simulink model "SingleTrack"  (R2019b)
settings: Solver=ode1  StartTime=0  StopTime=250  FixedStep=1.0000000000000000e-003  RelTol=1e-3
InitFcn:
  | sampleTime = str2double(get_param(bdroot, 'FixedStep'));
undefined symbols (not defined in the file or in its folder): AccPedalPos, BrakePedalPos, BrakeSwitch, DiscIntNeverNeededParam, DYNA4, EngSpd, IgnitionSwitch, InitialGear, InitialSpeed, IntendedEngTrq, LeftIndicator, MainBrakePress, MaxGear, MDL, MinGear, RefAcc, RefLane, RefLatPos, RefPath, RefPathCurv, RefSpd, RefSpdPreview, RefSpdRetrospect, RightIndicator, SteeringWheelAng, SteeringWheelTrq, UserDefinedRefValue, vm_const
libraries: UtilitiesLibrary x31, simulink x18, WheelSystemModules x13, LongitudinalControllerModules x13, LateralControllerModules x7, AnimationBusselectorModules x5, EnvironmentModules x5, BasicEngineControlModules x5, MiscellaneousControlModules x5, Animation3Modules x4, AuxiliariesModules x4, ReducedTireModules x4
(part 3 of 32)

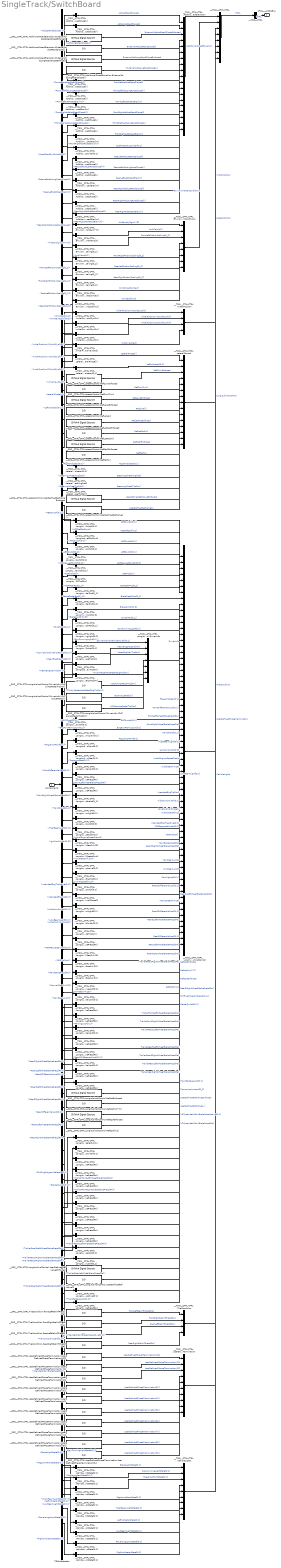
== system SingleTrack/SwitchBoard ==
  Components : Inport
  TDBusSelector : BusSelector  OutputSignals=Environment.AdditionalRoadElevation.AddLatRoadSlope[-],Environment.AdditionalRoadElevation.AddLongRoadSlope[-],Environment.AdditionalRoadElevation.FrontLeftAddLatRoadSlope[-],Environment.AdditionalRoadElevation.FrontLeftAddLongRoadSlope[-],Environment.AdditionalRoadElevation.FrontLeftAddRoadElev[m],Environment.AdditionalRoadElevation.FrontRightAddLatRoadSlope[-],Environment.AdditionalRoadElevation.FrontRightAddLongRoadSlope[-],Environment.AdditionalRoadElevation.FrontRightAddRoadElev[m],Environment.AdditionalRoadElevation.LocalRoadSysSwitch[0;1],Environment.AdditionalRoadElevation.RearLeftAddLatRoadSlope[-],Environment.AdditionalRoadElevation.RearLeftAddLongRoadSlope[-],Environment.AdditionalRoadElevation.RearLeftAddRoadElev[m],Environment.AdditionalRoadElevation.RearRightAddLatRoadSlope[-],Environment.AdditionalRoadElevation.RearRightAddLongRoadSlope[-],Environment.AdditionalRoadElevation.RearRightAddRoadElev[m],Environment.AmbientConditions.AirDensity[kg/m**3],Environment.AmbientConditions.AmbTemp[K],Environment.RoadFrictionScaling.FrontLeftFrictionScaling[0_2],Environment.RoadFrictionScaling.FrontRightFrictionScaling[0_2],Environment.RoadFrictionScaling.RearLeftFrictionScaling[0_2],Environment.RoadFrictionScaling.RearRightFrictionScaling[0_2],Environment.WindImpact.WindDirection[rad],Environment.WindImpact.WindSpd[m/s],VehicleControl.InitialConditions.InitialPositionX(WorldSys)[m],VehicleControl.InitialConditions.InitialPositionY(WorldSys)[m],VehicleControl.InitialConditions.InitialPositionZ(WorldSys)[m],VehicleControl.InitialConditions.InitialYaw[rad],VehicleControl.LateralControl.LateralPhase[-],VehicleControl.LateralControl.LeftIndicator[0;1],VehicleControl.LateralControl.RightIndicator[0;1],VehicleControl.LateralControl.SteeringWheelAng[rad],Vehicle.Chassis.FrontAxle.Steering.SteeringWheelTrq[Nm],VehicleControl.LongitudinalControl.ABSSwitch[0;1],VehicleControl.LongitudinalControl.ACCRefSpd[m/s],VehicleControl.LongitudinalControl.ACCSwitch[0;1],VehicleControl.LongitudinalControl.AEBSwitch[0;1],Vehicle.Drivetrain.DrivetrainControlUnit.TransmissionControlUnit.ASRRequestSwitch[0;2],Vehicle.Drivetrain.DrivetrainControlUnit.TransmissionControlUnit.ASRTrq[Nm],VehicleControl.LongitudinalControl.AccPedalPos[0_1],VehicleControl.LongitudinalControl.BrakePedalPos[0_1],VehicleControl.LongitudinalControl.BrakeSwitch[1;3],VehicleControl.LongitudinalControl.ClutchPos[0_1],VehicleControl.LongitudinalControl.DayRunningLight[0;1],ControlUnits.VCU.DriverInfo.ConventionalVehicleSwitch[0;1],Vehicle.Engine.EnginePhysics.Mechanics.MeanEngDragTrq[Nm],Vehicle.Engine.EnginePhysics.Mechanics.MeanEngMaxTrq[Nm],Vehicle.Engine.EnginePhysics.Mechanics.ThirtyPercentAccPedalEngTrq[Nm],VehicleControl.LongitudinalControl.ESCSwitch[0;1],ControlUnits.VCU.EngRunPermission[0;1],VehicleControl.LongitudinalControl.FogLampFront[0;1],VehicleControl.LongitudinalControl.FogLampRear[0;1],VehicleControl.LongitudinalControl.FrontDifferentialLock[0;1],VehicleControl.LongitudinalControl.FrontLeftWheelBrakePress[Pa],VehicleControl.LongitudinalControl.FrontRightWheelBrakePress[Pa],VehicleControl.LongitudinalControl.Handbrake[0_1],VehicleControl.LongitudinalControl.HighBeamLight[0;1],VehicleControl.LongitudinalControl.IgnitionSwitch[0;3],VehicleControl.LongitudinalControl.InitialEngineSpeed[rad/s],VehicleControl.LongitudinalControl.InitialGear[-4;20],VehicleControl.LongitudinalControl.InitialSpeed[m/s],ControlUnits.VCU.IntendedEngTrqActive[0;1],ControlUnits.VCU.IntendedEngTrq[Nm],VehicleControl.LongitudinalControl.KickdownSwitch[0;1],VehicleControl.LongitudinalControl.LongitudinalPhase[-],VehicleControl.LongitudinalControl.LowBeamLight[0;1],Vehicle.Drivetrain.DrivetrainControlUnit.TransmissionControlUnit.MSRRequestSwitch[0;2],Vehicle.Drivetrain.DrivetrainControlUnit.TransmissionControlUnit.MSRTrq[Nm],VehicleControl.LongitudinalControl.MainBrakePress[Pa],VehicleControl.LongitudinalControl.ManualGear[-4;20],VehicleControl.LongitudinalControl.AutomaticGearRange.MaxGear[-4;20],VehicleControl.LongitudinalControl.AutomaticGearRange.MinGear[-4;20],VehicleControl.LongitudinalControl.ParkingLock[0;1],VehicleControl.LongitudinalControl.Rear2DifferentialLock[0;1],VehicleControl.LongitudinalControl.Rear2LeftWheelBrakePress[Pa],VehicleControl.LongitudinalControl.Rear2RightWheelBrakePress[Pa],VehicleControl.LongitudinalControl.Rear3DifferentialLock[0;1],VehicleControl.LongitudinalControl.Rear3LeftWheelBrakePress[Pa],VehicleControl.LongitudinalControl.Rear3RightWheelBrakePress[Pa],VehicleControl.LongitudinalControl.RearDifferentialLock[0;1],VehicleControl.LongitudinalControl.RearLeftWheelBrakePress[Pa],VehicleControl.LongitudinalControl.RearRightWheelBrakePress[Pa],VehicleControl.LongitudinalControl.ShiftingProgramSelection[-],Vehicle.Engine.EngineControlUnit.StarterSwitch[0;1],VehicleControl.LongitudinalControl.TrailerFrontLeftWheelBrakePress[Pa],VehicleControl.LongitudinalControl.TrailerFrontRightWheelBrakePress[Pa],VehicleControl.LongitudinalControl.TrailerRear2LeftWheelBrakePress[Pa],VehicleControl.LongitudinalControl.TrailerRear2RightWheelBrakePress[Pa],VehicleControl.LongitudinalControl.TrailerRear3LeftWheelBrakePress[Pa],VehicleControl.LongitudinalControl.TrailerRear3RightWheelBrakePress[Pa],VehicleControl.LongitudinalControl.TrailerRearLeftWheelBrakePress[Pa],VehicleControl.LongitudinalControl.TrailerRearRightWheelBrakePress[Pa],VehicleControl.LongitudinalControl.TransferCaseLock[0;1],ControlUnits.VCU.TransmissionLoad[0_1],ControlUnits.VCU.IntendedMainBrakePressActive[0;1],ControlUnits.VCU.IntendedMainBrakePress[Pa],ControlUnits.LCU.VehicleLights.BrakeLightState[0;1],ControlUnits.LCU.VehicleLights.DayRunningLightState[0;1],ControlUnits.LCU.VehicleLights.FogLampFrontState[0;1],ControlUnits.LCU.VehicleLights.FogLampRearState[0;1],ControlUnits.LCU.VehicleLights.HighBeamLightState[0;1],ControlUnits.LCU.VehicleLights.LeftIndicatorState[0;1],ControlUnits.LCU.VehicleLights.LowBeamLightState[0;1],ControlUnits.LCU.VehicleLights.ReversingLampState[0;1],ControlUnits.LCU.VehicleLights.RightIndicatorState[0;1]
  __SRC__CTRL.CTRL.AdditionalRoadElevation.ExternalAddLatRoadSlopeEnforced : UtilitiesLibrary/DYNA4 Signal Source  Tag=DYNA4_Signal_Source  accessId=DYNA4.ModelHandling.AccessID.format('CTRL.AdditionalRoadElevation.ExternalAddLatRoadSlopeEnforced', 'parentId', parentId, 'blockName', blockName)  initialValue=0.0  sampleTime=sampleTime
  __SRC__CTRL.CTRL.AdditionalRoadElevation.ExternalAddLatRoadSlope[-] : Constant  Value=0.0  OutDataTypeStr=Inherit: Inherit via back propagation
  __SRC__CTRL.CTRL.AdditionalRoadElevation.ExternalAddLongRoadSlopeEnforced : UtilitiesLibrary/DYNA4 Signal Source  Tag=DYNA4_Signal_Source  accessId=DYNA4.ModelHandling.AccessID.format('CTRL.AdditionalRoadElevation.ExternalAddLongRoadSlopeEnforced', 'parentId', parentId, 'blockName', blockName)  initialValue=0.0  sampleTime=sampleTime
  __SRC__CTRL.CTRL.AdditionalRoadElevation.ExternalAddLongRoadSlope[-] : Constant  Value=0.0  OutDataTypeStr=Inherit: Inherit via back propagation
  __SRC__CTRL.CTRL.LateralControl.RefCurvEnforced : UtilitiesLibrary/DYNA4 Signal Source  Tag=DYNA4_Signal_Source  accessId=DYNA4.ModelHandling.AccessID.format('CTRL.LateralControl.RefCurvEnforced', 'parentId', parentId, 'blockName', blockName)  initialValue=0.0  sampleTime=sampleTime
  __SRC__CTRL.CTRL.LateralControl.RefCurv[1/m] : Constant  Value=0.0  OutDataTypeStr=Inherit: Inherit via back propagation
  __SRC__CTRL.CTRL.LateralControl.RefLaneEnforced : UtilitiesLibrary/DYNA4 Signal Source  Tag=DYNA4_Signal_Source  accessId=DYNA4.ModelHandling.AccessID.format('CTRL.LateralControl.RefLaneEnforced', 'parentId', parentId, 'blockName', blockName)  initialValue=0.0  sampleTime=sampleTime
  __SRC__CTRL.CTRL.LateralControl.RefLane[-] : Constant  Value=0.0  OutDataTypeStr=Inherit: Inherit via back propagation
  __SRC__CTRL.CTRL.LateralControl.RefLatPosEnforced : UtilitiesLibrary/DYNA4 Signal Source  Tag=DYNA4_Signal_Source  accessId=DYNA4.ModelHandling.AccessID.format('CTRL.LateralControl.RefLatPosEnforced', 'parentId', parentId, 'blockName', blockName)  initialValue=0.0  sampleTime=sampleTime
  __SRC__CTRL.CTRL.LateralControl.RefLatPos[m] : Constant  Value=0.0  OutDataTypeStr=Inherit: Inherit via back propagation
  __SRC__CTRL.CTRL.LateralControl.RefPathEnforced : UtilitiesLibrary/DYNA4 Signal Source  Tag=DYNA4_Signal_Source  accessId=DYNA4.ModelHandling.AccessID.format('CTRL.LateralControl.RefPathEnforced', 'parentId', parentId, 'blockName', blockName)  initialValue=0.0  sampleTime=sampleTime
  __SRC__CTRL.CTRL.LateralControl.RefPath[-] : Constant  Value=0.0  OutDataTypeStr=Inherit: Inherit via back propagation
  __SRC__CTRL.CTRL.LateralControl.UserDefinedRefValueEnforced : UtilitiesLibrary/DYNA4 Signal Source  Tag=DYNA4_Signal_Source  accessId=DYNA4.ModelHandling.AccessID.format('CTRL.LateralControl.UserDefinedRefValueEnforced', 'parentId', parentId, 'blockName', blockName)  initialValue=0.0  sampleTime=sampleTime
  __SRC__CTRL.CTRL.LateralControl.UserDefinedRefValue[-] : Constant  Value=0.0  OutDataTypeStr=Inherit: Inherit via back propagation
  __SRC__CTRL.CTRL.LongitudinalControl.DriverInfo.VCUFullAccPedalTrq[Nm] : Constant  Value=0.0  OutDataTypeStr=Inherit: Inherit via back propagation
  __SRC__CTRL.CTRL.LongitudinalControl.DriverInfo.VCUTorqueRatio[-] : Constant  Value=0.0  OutDataTypeStr=Inherit: Inherit via back propagation
  __SRC__CTRL.CTRL.LongitudinalControl.DriverInfo.VCUZeroAccPedalTrq[Nm] : Constant  Value=0.0  OutDataTypeStr=Inherit: Inherit via back propagation
  __SRC__CTRL.CTRL.LongitudinalControl.RefAccEnforced : UtilitiesLibrary/DYNA4 Signal Source  Tag=DYNA4_Signal_Source  accessId=DYNA4.ModelHandling.AccessID.format('CTRL.LongitudinalControl.RefAccEnforced', 'parentId', parentId, 'blockName', blockName)  initialValue=0.0  sampleTime=sampleTime
  __SRC__CTRL.CTRL.LongitudinalControl.RefAcc[m/s**2] : Constant  Value=0.0  OutDataTypeStr=Inherit: Inherit via back propagation
  __SRC__CTRL.CTRL.LongitudinalControl.RefSpdEnforced : UtilitiesLibrary/DYNA4 Signal Source  Tag=DYNA4_Signal_Source  accessId=DYNA4.ModelHandling.AccessID.format('CTRL.LongitudinalControl.RefSpdEnforced', 'parentId', parentId, 'blockName', blockName)  initialValue=0.0  sampleTime=sampleTime
  __SRC__CTRL.CTRL.LongitudinalControl.RefSpd[m/s] : Constant  Value=0.0  OutDataTypeStr=Inherit: Inherit via back propagation
  __SRC__CTRL.CTRL.LongitudinalControl.UserDefinedRefValueEnforced : UtilitiesLibrary/DYNA4 Signal Source  Tag=DYNA4_Signal_Source  accessId=DYNA4.ModelHandling.AccessID.format('CTRL.LongitudinalControl.UserDefinedRefValueEnforced', 'parentId', parentId, 'blockName', blockName)  initialValue=0.0  sampleTime=sampleTime
  __SRC__CTRL.CTRL.LongitudinalControl.UserDefinedRefValue[-] : Constant  Value=0.0  OutDataTypeStr=Inherit: Inherit via back propagation
  __SRC__CTRL.CTRL.TireCondition.FrontLeftRelInflPress[Pa] : Constant  Value=0.0  OutDataTypeStr=Inherit: Inherit via back propagation
  __SRC__CTRL.CTRL.TireCondition.FrontRightRelInflPress[Pa] : Constant  Value=0.0  OutDataTypeStr=Inherit: Inherit via back propagation
  __SRC__CTRL.CTRL.TireCondition.RearLeftRelInflPress[Pa] : Constant  Value=0.0  OutDataTypeStr=Inherit: Inherit via back propagation
  __SRC__CTRL.CTRL.TireCondition.RearRightRelInflPress[Pa] : Constant  Value=0.0  OutDataTypeStr=Inherit: Inherit via back propagation
  __SRC__CTRL.CTRL.UserDefinedPhaseTermination.UserDefinedPhaseTermination10[-] : Constant  Value=0.0  OutDataTypeStr=Inherit: Inherit via back propagation
  __SRC__CTRL.CTRL.UserDefinedPhaseTermination.UserDefinedPhaseTermination1[-] : Constant  Value=0.0  OutDataTypeStr=Inherit: Inherit via back propagation
  __SRC__CTRL.CTRL.UserDefinedPhaseTermination.UserDefinedPhaseTermination2[-] : Constant  Value=0.0  OutDataTypeStr=Inherit: Inherit via back propagation
  __SRC__CTRL.CTRL.UserDefinedPhaseTermination.UserDefinedPhaseTermination3[-] : Constant  Value=0.0  OutDataTypeStr=Inherit: Inherit via back propagation
  __SRC__CTRL.CTRL.UserDefinedPhaseTermination.UserDefinedPhaseTermination4[-] : Constant  Value=0.0  OutDataTypeStr=Inherit: Inherit via back propagation
  __SRC__CTRL.CTRL.UserDefinedPhaseTermination.UserDefinedPhaseTermination5[-] : Constant  Value=0.0  OutDataTypeStr=Inherit: Inherit via back propagation
  __SRC__CTRL.CTRL.UserDefinedPhaseTermination.UserDefinedPhaseTermination6[-] : Constant  Value=0.0  OutDataTypeStr=Inherit: Inherit via back propagation
  __SRC__CTRL.CTRL.UserDefinedPhaseTermination.UserDefinedPhaseTermination7[-] : Constant  Value=0.0  OutDataTypeStr=Inherit: Inherit via back propagation
  __SRC__CTRL.CTRL.UserDefinedPhaseTermination.UserDefinedPhaseTermination8[-] : Constant  Value=0.0  OutDataTypeStr=Inherit: Inherit via back propagation
  __SRC__CTRL.CTRL.UserDefinedPhaseTermination.UserDefinedPhaseTermination9[-] : Constant  Value=0.0  OutDataTypeStr=Inherit: Inherit via back propagation
  __TDD__CTRL.CTRL.AdditionalRoadElevation.AddLatRoadSlope[-] : Demux  Outputs=[1]
  __TDD__CTRL.CTRL.AdditionalRoadElevation.AddLongRoadSlope[-] : Demux  Outputs=[1]
  __TDD__CTRL.CTRL.AdditionalRoadElevation.FrontLeftAddLatRoadSlope[-] : Demux  Outputs=[1]
  __TDD__CTRL.CTRL.AdditionalRoadElevation.FrontLeftAddLongRoadSlope[-] : Demux  Outputs=[1]
  __TDD__CTRL.CTRL.AdditionalRoadElevation.FrontLeftAddRoadElev[m] : Demux  Outputs=[1]
  __TDD__CTRL.CTRL.AdditionalRoadElevation.FrontRightAddLatRoadSlope[-] : Demux  Outputs=[1]
  __TDD__CTRL.CTRL.AdditionalRoadElevation.FrontRightAddLongRoadSlope[-] : Demux  Outputs=[1]
  __TDD__CTRL.CTRL.AdditionalRoadElevation.FrontRightAddRoadElev[m] : Demux  Outputs=[1]
  __TDD__CTRL.CTRL.AdditionalRoadElevation.LocalRoadSysSwitch[0;1] : Demux  Outputs=[1]
  __TDD__CTRL.CTRL.AdditionalRoadElevation.RearLeftAddLatRoadSlope[-] : Demux  Outputs=[1]
  __TDD__CTRL.CTRL.AdditionalRoadElevation.RearLeftAddLongRoadSlope[-] : Demux  Outputs=[1]
  __TDD__CTRL.CTRL.AdditionalRoadElevation.RearLeftAddRoadElev[m] : Demux  Outputs=[1]
  __TDD__CTRL.CTRL.AdditionalRoadElevation.RearRightAddLatRoadSlope[-] : Demux  Outputs=[1]
  __TDD__CTRL.CTRL.AdditionalRoadElevation.RearRightAddLongRoadSlope[-] : Demux  Outputs=[1]
  __TDD__CTRL.CTRL.AdditionalRoadElevation.RearRightAddRoadElev[m] : Demux  Outputs=[1]
  __TDD__CTRL.CTRL.EnvironmentalConditions.AirDensity[kg/m**3] : Demux  Outputs=[1]
  __TDD__CTRL.CTRL.EnvironmentalConditions.AmbTemp[K] : Demux  Outputs=[1]
  __TDD__CTRL.CTRL.EnvironmentalConditions.FrontLeftFrictionScaling[0_2] : Demux  Outputs=[1]
  __TDD__CTRL.CTRL.EnvironmentalConditions.FrontRightFrictionScaling[0_2] : Demux  Outputs=[1]
  __TDD__CTRL.CTRL.EnvironmentalConditions.RearLeftFrictionScaling[0_2] : Demux  Outputs=[1]
  __TDD__CTRL.CTRL.EnvironmentalConditions.RearRightFrictionScaling[0_2] : Demux  Outputs=[1]
  __TDD__CTRL.CTRL.EnvironmentalConditions.WindDirection[rad] : Demux  Outputs=[1]
  __TDD__CTRL.CTRL.EnvironmentalConditions.WindSpd[m/s] : Demux  Outputs=[1]
  __TDD__CTRL.CTRL.InitialPosition.InitialPositionX(WorldSys)[m] : Demux  Outputs=[1]
  __TDD__CTRL.CTRL.InitialPosition.InitialPositionY(WorldSys)[m] : Demux  Outputs=[1]
  __TDD__CTRL.CTRL.InitialPosition.InitialPositionZ(WorldSys)[m] : Demux  Outputs=[1]
  __TDD__CTRL.CTRL.InitialPosition.InitialYaw[rad] : Demux  Outputs=[1]
  __TDD__CTRL.CTRL.LateralControl.LateralPhase[-] : Demux  Outputs=1
  __TDD__CTRL.CTRL.LateralControl.LeftIndicator[0;1] : Demux  Outputs=[1]
  __TDD__CTRL.CTRL.LateralControl.RightIndicator[0;1] : Demux  Outputs=[1]
  __TDD__CTRL.CTRL.LateralControl.SteeringWheelAng[rad] : Demux  Outputs=[1]
  __TDD__CTRL.CTRL.LateralControl.SteeringWheelTrq[Nm] : Demux  Outputs=[1]
  __TDD__CTRL.CTRL.LongitudinalControl.ABSSwitch[0;1] : Demux  Outputs=[1]
  __TDD__CTRL.CTRL.LongitudinalControl.ACCRefSpd[m/s] : Demux  Outputs=[1]
  __TDD__CTRL.CTRL.LongitudinalControl.ACCSwitch[0;1] : Demux  Outputs=[1]
  __TDD__CTRL.CTRL.LongitudinalControl.AEBSwitch[0;1] : Demux  Outputs=[1]
  __TDD__CTRL.CTRL.LongitudinalControl.ASRRequestSwitch[0;2] : Demux  Outputs=1
  __TDD__CTRL.CTRL.LongitudinalControl.ASRTrq[Nm] : Demux  Outputs=1
  __TDD__CTRL.CTRL.LongitudinalControl.AccPedalPos[0_1] : Demux  Outputs=[1]
  __TDD__CTRL.CTRL.LongitudinalControl.BrakePedalPos[0_1] : Demux  Outputs=1
  __TDD__CTRL.CTRL.LongitudinalControl.BrakeSwitch[1;3] : Demux  Outputs=1
  __TDD__CTRL.CTRL.LongitudinalControl.ClutchPos[0_1] : Demux  Outputs=[1]
  __TDD__CTRL.CTRL.LongitudinalControl.DayRunningLight[0;1] : Demux  Outputs=[1]
  __TDD__CTRL.CTRL.LongitudinalControl.DriverInfo.ConventionalVehicleSwitch[0;1] : Demux  Outputs=[1]
  __TDD__CTRL.CTRL.LongitudinalControl.DriverInfo.MeanEngDragTrq[Nm] : Demux  Outputs=[1]
  __TDD__CTRL.CTRL.LongitudinalControl.DriverInfo.MeanEngMaxTrq[Nm] : Demux  Outputs=[1]
  __TDD__CTRL.CTRL.LongitudinalControl.DriverInfo.ThirtyPercentAccPedalEngTrq[Nm] : Demux  Outputs=[1]
  __TDD__CTRL.CTRL.LongitudinalControl.ESCSwitch[0;1] : Demux  Outputs=[1]
  __TDD__CTRL.CTRL.LongitudinalControl.EngRunPermission[0;1] : Demux  Outputs=[1]
  __TDD__CTRL.CTRL.LongitudinalControl.FogLampFront[0;1] : Demux  Outputs=[1]
  __TDD__CTRL.CTRL.LongitudinalControl.FogLampRear[0;1] : Demux  Outputs=[1]
  __TDD__CTRL.CTRL.LongitudinalControl.FrontDifferentialLock[0;1] : Demux  Outputs=[1]
  __TDD__CTRL.CTRL.LongitudinalControl.FrontLeftWheelBrakePress[Pa] : Demux  Outputs=1
  __TDD__CTRL.CTRL.LongitudinalControl.FrontRightWheelBrakePress[Pa] : Demux  Outputs=1
  __TDD__CTRL.CTRL.LongitudinalControl.Handbrake[0_1] : Demux  Outputs=[1]
  __TDD__CTRL.CTRL.LongitudinalControl.HighBeamLight[0;1] : Demux  Outputs=[1]
  __TDD__CTRL.CTRL.LongitudinalControl.IgnitionSwitch[0;3] : Demux  Outputs=1
  __TDD__CTRL.CTRL.LongitudinalControl.InitialEngineSpeed[rad/s] : Demux  Outputs=[1]
  __TDD__CTRL.CTRL.LongitudinalControl.InitialGear[-4;20] : Demux  Outputs=[1]
  __TDD__CTRL.CTRL.LongitudinalControl.InitialSpeed[m/s] : Demux  Outputs=[1]
  __TDD__CTRL.CTRL.LongitudinalControl.IntendedEngTrqActive[0;1] : Demux  Outputs=[1]
  __TDD__CTRL.CTRL.LongitudinalControl.IntendedEngTrq[Nm] : Demux  Outputs=[1]
  __TDD__CTRL.CTRL.LongitudinalControl.KickdownSwitch[0;1] : Demux  Outputs=[1]
  __TDD__CTRL.CTRL.LongitudinalControl.LongitudinalPhase[-] : Demux  Outputs=1
  __TDD__CTRL.CTRL.LongitudinalControl.LowBeamLight[0;1] : Demux  Outputs=[1]
  __TDD__CTRL.CTRL.LongitudinalControl.MSRRequestSwitch[0;2] : Demux  Outputs=1
  __TDD__CTRL.CTRL.LongitudinalControl.MSRTrq[Nm] : Demux  Outputs=1
  __TDD__CTRL.CTRL.LongitudinalControl.MainBrakePress[Pa] : Demux  Outputs=1
  __TDD__CTRL.CTRL.LongitudinalControl.ManualGear[-4;20] : Demux  Outputs=[1]
  __TDD__CTRL.CTRL.LongitudinalControl.MaxGear[-4;20] : Demux  Outputs=[1]
  __TDD__CTRL.CTRL.LongitudinalControl.MinGear[-4;20] : Demux  Outputs=[1]
  __TDD__CTRL.CTRL.LongitudinalControl.ParkingLock[0;1] : Demux  Outputs=[1]
  __TDD__CTRL.CTRL.LongitudinalControl.Rear2DifferentialLock[0;1] : Demux  Outputs=[1]
  __TDD__CTRL.CTRL.LongitudinalControl.Rear2LeftWheelBrakePress[Pa] : Demux  Outputs=1
  __TDD__CTRL.CTRL.LongitudinalControl.Rear2RightWheelBrakePress[Pa] : Demux  Outputs=1
  __TDD__CTRL.CTRL.LongitudinalControl.Rear3DifferentialLock[0;1] : Demux  Outputs=[1]
  __TDD__CTRL.CTRL.LongitudinalControl.Rear3LeftWheelBrakePress[Pa] : Demux  Outputs=1
  __TDD__CTRL.CTRL.LongitudinalControl.Rear3RightWheelBrakePress[Pa] : Demux  Outputs=1
  __TDD__CTRL.CTRL.LongitudinalControl.RearDifferentialLock[0;1] : Demux  Outputs=[1]
  __TDD__CTRL.CTRL.LongitudinalControl.RearLeftWheelBrakePress[Pa] : Demux  Outputs=1
  __TDD__CTRL.CTRL.LongitudinalControl.RearRightWheelBrakePress[Pa] : Demux  Outputs=1
  __TDD__CTRL.CTRL.LongitudinalControl.ShiftingProgramSelection[-] : Demux  Outputs=[1]
  __TDD__CTRL.CTRL.LongitudinalControl.StarterSwitch[0;1] : Demux  Outputs=[1]
  __TDD__CTRL.CTRL.LongitudinalControl.TrailerFrontLeftWheelBrakePress[Pa] : Demux  Outputs=[1]
  __TDD__CTRL.CTRL.LongitudinalControl.TrailerFrontRightWheelBrakePress[Pa] : Demux  Outputs=[1]
  __TDD__CTRL.CTRL.LongitudinalControl.TrailerRear2LeftWheelBrakePress[Pa] : Demux  Outputs=[1]
  __TDD__CTRL.CTRL.LongitudinalControl.TrailerRear2RightWheelBrakePress[Pa] : Demux  Outputs=[1]
  __TDD__CTRL.CTRL.LongitudinalControl.TrailerRear3LeftWheelBrakePress[Pa] : Demux  Outputs=[1]
  __TDD__CTRL.CTRL.LongitudinalControl.TrailerRear3RightWheelBrakePress[Pa] : Demux  Outputs=[1]
  __TDD__CTRL.CTRL.LongitudinalControl.TrailerRearLeftWheelBrakePress[Pa] : Demux  Outputs=[1]
  __TDD__CTRL.CTRL.LongitudinalControl.TrailerRearRightWheelBrakePress[Pa] : Demux  Outputs=[1]
  __TDD__CTRL.CTRL.LongitudinalControl.TransferCaseLock[0;1] : Demux  Outputs=[1]
  __TDD__CTRL.CTRL.LongitudinalControl.TransmissionLoad[0_1] : Demux  Outputs=[1]
  __TDD__CTRL.CTRL.LongitudinalControl.VCUIntendedMainBrakePressActive[0;1] : Demux  Outputs=[1]
  __TDD__CTRL.CTRL.LongitudinalControl.VCUIntendedMainBrakePress[Pa] : Demux  Outputs=[1]
  __TDD__CTRL.CTRL.VehicleLights.BrakeLightState[0;1] : Demux  Outputs=1
  __TDD__CTRL.CTRL.VehicleLights.DayRunningLightState[0;1] : Demux  Outputs=1
  __TDD__CTRL.CTRL.VehicleLights.FogLampFrontState[0;1] : Demux  Outputs=1
  __TDD__CTRL.CTRL.VehicleLights.FogLampRearState[0;1] : Demux  Outputs=1
  __TDD__CTRL.CTRL.VehicleLights.HighBeamLightState[0;1] : Demux  Outputs=1
  __TDD__CTRL.CTRL.VehicleLights.LeftIndicatorState[0;1] : Demux  Outputs=1
  __TDD__CTRL.CTRL.VehicleLights.LowBeamLightState[0;1] : Demux  Outputs=1
  __TDD__CTRL.CTRL.VehicleLights.ReversingLampState[0;1] : Demux  Outputs=1
  __TDD__CTRL.CTRL.VehicleLights.RightIndicatorState[0;1] : Demux  Outputs=1
  __TDO__CTRL : BusCreator  Inputs=1
  __TDO__CTRL.CTRL : BusCreator  Inputs=8
  __TDO__CTRL.CTRL.AdditionalRoadElevation : BusCreator  Inputs=19
  __TDO__CTRL.CTRL.EnvironmentalConditions : BusCreator  Inputs=8
  __TDO__CTRL.CTRL.InitialPosition : BusCreator  Inputs=4
  __TDO__CTRL.CTRL.LateralControl : BusCreator  Inputs=15
  __TDO__CTRL.CTRL.LongitudinalControl : BusCreator  Inputs=66
  __TDO__CTRL.CTRL.LongitudinalControl.DriverInfo : BusCreator  Inputs=7
  __TDO__CTRL.CTRL.TireCondition : BusCreator  Inputs=4
  __TDO__CTRL.CTRL.UserDefinedPhaseTermination : BusCreator  Inputs=10
  __TDO__CTRL.CTRL.VehicleLights : BusCreator  Inputs=9
  CTRL___UNIQUE_1 : Outport  Description=|  VectorParamsAs1DForOutWhenUnconnected=off
      | <name>Environment.AdditionalRoadElevation.AddLatRoadSlope[-]</name>
      | <comment></comment>
  wires:
  Components/1 -> TDBusSelector/1
  TDBusSelector/1 -> __TDD__CTRL.CTRL.AdditionalRoadElevation.AddLatRoadSlope[-]/1  "<AddLatRoadSlope[-]>"
  __TDD__CTRL.CTRL.AdditionalRoadElevation.AddLatRoadSlope[-]/1 -> __TDO__CTRL.CTRL.AdditionalRoadElevation/1  "AddLatRoadSlope[-]"
  __TDO__CTRL.CTRL.AdditionalRoadElevation/1 -> __TDO__CTRL.CTRL/1  "AdditionalRoadElevation"
  __TDO__CTRL.CTRL/1 -> __TDO__CTRL/1  "CTRL"
  TDBusSelector/2 -> __TDD__CTRL.CTRL.AdditionalRoadElevation.AddLongRoadSlope[-]/1  "<AddLongRoadSlope[-]>"
  __TDD__CTRL.CTRL.AdditionalRoadElevation.AddLongRoadSlope[-]/1 -> __TDO__CTRL.CTRL.AdditionalRoadElevation/2  "AddLongRoadSlope[-]"
  __SRC__CTRL.CTRL.AdditionalRoadElevation.ExternalAddLatRoadSlopeEnforced/1 -> __TDO__CTRL.CTRL.AdditionalRoadElevation/3  "ExternalAddLatRoadSlopeEnforced"
  __SRC__CTRL.CTRL.AdditionalRoadElevation.ExternalAddLatRoadSlope[-]/1 -> __TDO__CTRL.CTRL.AdditionalRoadElevation/4  "ExternalAddLatRoadSlope[-]"
  __SRC__CTRL.CTRL.AdditionalRoadElevation.ExternalAddLongRoadSlopeEnforced/1 -> __TDO__CTRL.CTRL.AdditionalRoadElevation/5  "ExternalAddLongRoadSlopeEnforced"
  __SRC__CTRL.CTRL.AdditionalRoadElevation.ExternalAddLongRoadSlope[-]/1 -> __TDO__CTRL.CTRL.AdditionalRoadElevation/6  "ExternalAddLongRoadSlope[-]"
  TDBusSelector/3 -> __TDD__CTRL.CTRL.AdditionalRoadElevation.FrontLeftAddLatRoadSlope[-]/1  "<FrontLeftAddLatRoadSlope[-]>"
  __TDD__CTRL.CTRL.AdditionalRoadElevation.FrontLeftAddLatRoadSlope[-]/1 -> __TDO__CTRL.CTRL.AdditionalRoadElevation/7  "FrontLeftAddLatRoadSlope[-]"
  TDBusSelector/4 -> __TDD__CTRL.CTRL.AdditionalRoadElevation.FrontLeftAddLongRoadSlope[-]/1  "<FrontLeftAddLongRoadSlope[-]>"
  __TDD__CTRL.CTRL.AdditionalRoadElevation.FrontLeftAddLongRoadSlope[-]/1 -> __TDO__CTRL.CTRL.AdditionalRoadElevation/8  "FrontLeftAddLongRoadSlope[-]"
  TDBusSelector/5 -> __TDD__CTRL.CTRL.AdditionalRoadElevation.FrontLeftAddRoadElev[m]/1  "<FrontLeftAddRoadElev[m]>"
  __TDD__CTRL.CTRL.AdditionalRoadElevation.FrontLeftAddRoadElev[m]/1 -> __TDO__CTRL.CTRL.AdditionalRoadElevation/9  "FrontLeftAddRoadElev[m]"
  TDBusSelector/6 -> __TDD__CTRL.CTRL.AdditionalRoadElevation.FrontRightAddLatRoadSlope[-]/1  "<FrontRightAddLatRoadSlope[-]>"
  __TDD__CTRL.CTRL.AdditionalRoadElevation.FrontRightAddLatRoadSlope[-]/1 -> __TDO__CTRL.CTRL.AdditionalRoadElevation/10  "FrontRightAddLatRoadSlope[-]"
  TDBusSelector/7 -> __TDD__CTRL.CTRL.AdditionalRoadElevation.FrontRightAddLongRoadSlope[-]/1  "<FrontRightAddLongRoadSlope[-]>"
  __TDD__CTRL.CTRL.AdditionalRoadElevation.FrontRightAddLongRoadSlope[-]/1 -> __TDO__CTRL.CTRL.AdditionalRoadElevation/11  "FrontRightAddLongRoadSlope[-]"
  TDBusSelector/8 -> __TDD__CTRL.CTRL.AdditionalRoadElevation.FrontRightAddRoadElev[m]/1  "<FrontRightAddRoadElev[m]>"
  __TDD__CTRL.CTRL.AdditionalRoadElevation.FrontRightAddRoadElev[m]/1 -> __TDO__CTRL.CTRL.AdditionalRoadElevation/12  "FrontRightAddRoadElev[m]"
  TDBusSelector/9 -> __TDD__CTRL.CTRL.AdditionalRoadElevation.LocalRoadSysSwitch[0;1]/1  "<LocalRoadSysSwitch[0;1]>"
  __TDD__CTRL.CTRL.AdditionalRoadElevation.LocalRoadSysSwitch[0;1]/1 -> __TDO__CTRL.CTRL.AdditionalRoadElevation/13  "LocalRoadSysSwitch[0;1]"
  TDBusSelector/10 -> __TDD__CTRL.CTRL.AdditionalRoadElevation.RearLeftAddLatRoadSlope[-]/1  "<RearLeftAddLatRoadSlope[-]>"
  __TDD__CTRL.CTRL.AdditionalRoadElevation.RearLeftAddLatRoadSlope[-]/1 -> __TDO__CTRL.CTRL.AdditionalRoadElevation/14  "RearLeftAddLatRoadSlope[-]"
  TDBusSelector/11 -> __TDD__CTRL.CTRL.AdditionalRoadElevation.RearLeftAddLongRoadSlope[-]/1  "<RearLeftAddLongRoadSlope[-]>"
  __TDD__CTRL.CTRL.AdditionalRoadElevation.RearLeftAddLongRoadSlope[-]/1 -> __TDO__CTRL.CTRL.AdditionalRoadElevation/15  "RearLeftAddLongRoadSlope[-]"
  TDBusSelector/12 -> __TDD__CTRL.CTRL.AdditionalRoadElevation.RearLeftAddRoadElev[m]/1  "<RearLeftAddRoadElev[m]>"
  __TDD__CTRL.CTRL.AdditionalRoadElevation.RearLeftAddRoadElev[m]/1 -> __TDO__CTRL.CTRL.AdditionalRoadElevation/16  "RearLeftAddRoadElev[m]"
  TDBusSelector/13 -> __TDD__CTRL.CTRL.AdditionalRoadElevation.RearRightAddLatRoadSlope[-]/1  "<RearRightAddLatRoadSlope[-]>"
  __TDD__CTRL.CTRL.AdditionalRoadElevation.RearRightAddLatRoadSlope[-]/1 -> __TDO__CTRL.CTRL.AdditionalRoadElevation/17  "RearRightAddLatRoadSlope[-]"
  TDBusSelector/14 -> __TDD__CTRL.CTRL.AdditionalRoadElevation.RearRightAddLongRoadSlope[-]/1  "<RearRightAddLongRoadSlope[-]>"
  __TDD__CTRL.CTRL.AdditionalRoadElevation.RearRightAddLongRoadSlope[-]/1 -> __TDO__CTRL.CTRL.AdditionalRoadElevation/18  "RearRightAddLongRoadSlope[-]"
  TDBusSelector/15 -> __TDD__CTRL.CTRL.AdditionalRoadElevation.RearRightAddRoadElev[m]/1  "<RearRightAddRoadElev[m]>"
  __TDD__CTRL.CTRL.AdditionalRoadElevation.RearRightAddRoadElev[m]/1 -> __TDO__CTRL.CTRL.AdditionalRoadElevation/19  "RearRightAddRoadElev[m]"
  TDBusSelector/16 -> __TDD__CTRL.CTRL.EnvironmentalConditions.AirDensity[kg/m**3]/1  "<AirDensity[kg/m**3]>"
  __TDD__CTRL.CTRL.EnvironmentalConditions.AirDensity[kg/m**3]/1 -> __TDO__CTRL.CTRL.EnvironmentalConditions/1  "AirDensity[kg/m**3]"
  __TDO__CTRL.CTRL.EnvironmentalConditions/1 -> __TDO__CTRL.CTRL/2  "EnvironmentalConditions"
  TDBusSelector/17 -> __TDD__CTRL.CTRL.EnvironmentalConditions.AmbTemp[K]/1  "<AmbTemp[K]>"
  __TDD__CTRL.CTRL.EnvironmentalConditions.AmbTemp[K]/1 -> __TDO__CTRL.CTRL.EnvironmentalConditions/2  "AmbTemp[K]"
  TDBusSelector/18 -> __TDD__CTRL.CTRL.EnvironmentalConditions.FrontLeftFrictionScaling[0_2]/1  "<FrontLeftFrictionScaling[0_2]>"
  __TDD__CTRL.CTRL.EnvironmentalConditions.FrontLeftFrictionScaling[0_2]/1 -> __TDO__CTRL.CTRL.EnvironmentalConditions/3  "FrontLeftFrictionScaling[0_2]"
  TDBusSelector/19 -> __TDD__CTRL.CTRL.EnvironmentalConditions.FrontRightFrictionScaling[0_2]/1  "<FrontRightFrictionScaling[0_2]>"
  __TDD__CTRL.CTRL.EnvironmentalConditions.FrontRightFrictionScaling[0_2]/1 -> __TDO__CTRL.CTRL.EnvironmentalConditions/4  "FrontRightFrictionScaling[0_2]"
  TDBusSelector/20 -> __TDD__CTRL.CTRL.EnvironmentalConditions.RearLeftFrictionScaling[0_2]/1  "<RearLeftFrictionScaling[0_2]>"
  __TDD__CTRL.CTRL.EnvironmentalConditions.RearLeftFrictionScaling[0_2]/1 -> __TDO__CTRL.CTRL.EnvironmentalConditions/5  "RearLeftFrictionScaling[0_2]"
  TDBusSelector/21 -> __TDD__CTRL.CTRL.EnvironmentalConditions.RearRightFrictionScaling[0_2]/1  "<RearRightFrictionScaling[0_2]>"
  __TDD__CTRL.CTRL.EnvironmentalConditions.RearRightFrictionScaling[0_2]/1 -> __TDO__CTRL.CTRL.EnvironmentalConditions/6  "RearRightFrictionScaling[0_2]"
  TDBusSelector/22 -> __TDD__CTRL.CTRL.EnvironmentalConditions.WindDirection[rad]/1  "<WindDirection[rad]>"
  __TDD__CTRL.CTRL.EnvironmentalConditions.WindDirection[rad]/1 -> __TDO__CTRL.CTRL.EnvironmentalConditions/7  "WindDirection[rad]"
  TDBusSelector/23 -> __TDD__CTRL.CTRL.EnvironmentalConditions.WindSpd[m/s]/1  "<WindSpd[m/s]>"
  __TDD__CTRL.CTRL.EnvironmentalConditions.WindSpd[m/s]/1 -> __TDO__CTRL.CTRL.EnvironmentalConditions/8  "WindSpd[m/s]"
  TDBusSelector/24 -> __TDD__CTRL.CTRL.InitialPosition.InitialPositionX(WorldSys)[m]/1  "<InitialPositionX(WorldSys)[m]>"
  __TDD__CTRL.CTRL.InitialPosition.InitialPositionX(WorldSys)[m]/1 -> __TDO__CTRL.CTRL.InitialPosition/1  "InitialPositionX(WorldSys)[m]"
  __TDO__CTRL.CTRL.InitialPosition/1 -> __TDO__CTRL.CTRL/3  "InitialPosition"
  TDBusSelector/25 -> __TDD__CTRL.CTRL.InitialPosition.InitialPositionY(WorldSys)[m]/1  "<InitialPositionY(WorldSys)[m]>"
  __TDD__CTRL.CTRL.InitialPosition.InitialPositionY(WorldSys)[m]/1 -> __TDO__CTRL.CTRL.InitialPosition/2  "InitialPositionY(WorldSys)[m]"
  TDBusSelector/26 -> __TDD__CTRL.CTRL.InitialPosition.InitialPositionZ(WorldSys)[m]/1  "<InitialPositionZ(WorldSys)[m]>"
  __TDD__CTRL.CTRL.InitialPosition.InitialPositionZ(WorldSys)[m]/1 -> __TDO__CTRL.CTRL.InitialPosition/3  "InitialPositionZ(WorldSys)[m]"
  TDBusSelector/27 -> __TDD__CTRL.CTRL.InitialPosition.InitialYaw[rad]/1  "<InitialYaw[rad]>"
  __TDD__CTRL.CTRL.InitialPosition.InitialYaw[rad]/1 -> __TDO__CTRL.CTRL.InitialPosition/4  "InitialYaw[rad]"
  TDBusSelector/28 -> __TDD__CTRL.CTRL.LateralControl.LateralPhase[-]/1  "<LateralPhase[-]>"
  __TDD__CTRL.CTRL.LateralControl.LateralPhase[-]/1 -> __TDO__CTRL.CTRL.LateralControl/1  "LateralPhase[-]"
  __TDO__CTRL.CTRL.LateralControl/1 -> __TDO__CTRL.CTRL/4  "LateralControl"
  TDBusSelector/29 -> __TDD__CTRL.CTRL.LateralControl.LeftIndicator[0;1]/1  "<LeftIndicator[0;1]>"
  __TDD__CTRL.CTRL.LateralControl.LeftIndicator[0;1]/1 -> __TDO__CTRL.CTRL.LateralControl/2  "LeftIndicator[0;1]"
  __SRC__CTRL.CTRL.LateralControl.RefCurvEnforced/1 -> __TDO__CTRL.CTRL.LateralControl/3  "RefCurvEnforced"
  __SRC__CTRL.CTRL.LateralControl.RefCurv[1/m]/1 -> __TDO__CTRL.CTRL.LateralControl/4  "RefCurv[1/m]"
  __SRC__CTRL.CTRL.LateralControl.RefLaneEnforced/1 -> __TDO__CTRL.CTRL.LateralControl/5  "RefLaneEnforced"
  __SRC__CTRL.CTRL.LateralControl.RefLane[-]/1 -> __TDO__CTRL.CTRL.LateralControl/6  "RefLane[-]"
  __SRC__CTRL.CTRL.LateralControl.RefLatPosEnforced/1 -> __TDO__CTRL.CTRL.LateralControl/7  "RefLatPosEnforced"
  __SRC__CTRL.CTRL.LateralControl.RefLatPos[m]/1 -> __TDO__CTRL.CTRL.LateralControl/8  "RefLatPos[m]"
  __SRC__CTRL.CTRL.LateralControl.RefPathEnforced/1 -> __TDO__CTRL.CTRL.LateralControl/9  "RefPathEnforced"
  __SRC__CTRL.CTRL.LateralControl.RefPath[-]/1 -> __TDO__CTRL.CTRL.LateralControl/10  "RefPath[-]"
  TDBusSelector/30 -> __TDD__CTRL.CTRL.LateralControl.RightIndicator[0;1]/1  "<RightIndicator[0;1]>"
  __TDD__CTRL.CTRL.LateralControl.RightIndicator[0;1]/1 -> __TDO__CTRL.CTRL.LateralControl/11  "RightIndicator[0;1]"
  TDBusSelector/31 -> __TDD__CTRL.CTRL.LateralControl.SteeringWheelAng[rad]/1  "<SteeringWheelAng[rad]>"
  __TDD__CTRL.CTRL.LateralControl.SteeringWheelAng[rad]/1 -> __TDO__CTRL.CTRL.LateralControl/12  "SteeringWheelAng[rad]"
  TDBusSelector/32 -> __TDD__CTRL.CTRL.LateralControl.SteeringWheelTrq[Nm]/1  "<SteeringWheelTrq[Nm]>"
  __TDD__CTRL.CTRL.LateralControl.SteeringWheelTrq[Nm]/1 -> __TDO__CTRL.CTRL.LateralControl/13  "SteeringWheelTrq[Nm]"
  __SRC__CTRL.CTRL.LateralControl.UserDefinedRefValueEnforced/1 -> __TDO__CTRL.CTRL.LateralControl/14  "UserDefinedRefValueEnforced"
  __SRC__CTRL.CTRL.LateralControl.UserDefinedRefValue[-]/1 -> __TDO__CTRL.CTRL.LateralControl/15  "UserDefinedRefValue[-]"
  TDBusSelector/33 -> __TDD__CTRL.CTRL.LongitudinalControl.ABSSwitch[0;1]/1  "<ABSSwitch[0;1]>"
  __TDD__CTRL.CTRL.LongitudinalControl.ABSSwitch[0;1]/1 -> __TDO__CTRL.CTRL.LongitudinalControl/1  "ABSSwitch[0;1]"
  __TDO__CTRL.CTRL.LongitudinalControl/1 -> __TDO__CTRL.CTRL/5  "LongitudinalControl"
  TDBusSelector/34 -> __TDD__CTRL.CTRL.LongitudinalControl.ACCRefSpd[m/s]/1  "<ACCRefSpd[m/s]>"
  __TDD__CTRL.CTRL.LongitudinalControl.ACCRefSpd[m/s]/1 -> __TDO__CTRL.CTRL.LongitudinalControl/2  "ACCRefSpd[m/s]"
  TDBusSelector/35 -> __TDD__CTRL.CTRL.LongitudinalControl.ACCSwitch[0;1]/1  "<ACCSwitch[0;1]>"
  __TDD__CTRL.CTRL.LongitudinalControl.ACCSwitch[0;1]/1 -> __TDO__CTRL.CTRL.LongitudinalControl/3  "ACCSwitch[0;1]"
  TDBusSelector/36 -> __TDD__CTRL.CTRL.LongitudinalControl.AEBSwitch[0;1]/1  "<AEBSwitch[0;1]>"
  __TDD__CTRL.CTRL.LongitudinalControl.AEBSwitch[0;1]/1 -> __TDO__CTRL.CTRL.LongitudinalControl/4  "AEBSwitch[0;1]"
  TDBusSelector/37 -> __TDD__CTRL.CTRL.LongitudinalControl.ASRRequestSwitch[0;2]/1  "<ASRRequestSwitch[0;2]>"
  __TDD__CTRL.CTRL.LongitudinalControl.ASRRequestSwitch[0;2]/1 -> __TDO__CTRL.CTRL.LongitudinalControl/5  "ASRRequestSwitch[0;2]"
  TDBusSelector/38 -> __TDD__CTRL.CTRL.LongitudinalControl.ASRTrq[Nm]/1  "<ASRTrq[Nm]>"
  __TDD__CTRL.CTRL.LongitudinalControl.ASRTrq[Nm]/1 -> __TDO__CTRL.CTRL.LongitudinalControl/6  "ASRTrq[Nm]"
  TDBusSelector/39 -> __TDD__CTRL.CTRL.LongitudinalControl.AccPedalPos[0_1]/1  "<AccPedalPos[0_1]>"
  __TDD__CTRL.CTRL.LongitudinalControl.AccPedalPos[0_1]/1 -> __TDO__CTRL.CTRL.LongitudinalControl/7  "AccPedalPos[0_1]"
  TDBusSelector/40 -> __TDD__CTRL.CTRL.LongitudinalControl.BrakePedalPos[0_1]/1  "<BrakePedalPos[0_1]>"
  __TDD__CTRL.CTRL.LongitudinalControl.BrakePedalPos[0_1]/1 -> __TDO__CTRL.CTRL.LongitudinalControl/8  "BrakePedalPos[0_1]"
  TDBusSelector/41 -> __TDD__CTRL.CTRL.LongitudinalControl.BrakeSwitch[1;3]/1  "<BrakeSwitch[1;3]>"
  __TDD__CTRL.CTRL.LongitudinalControl.BrakeSwitch[1;3]/1 -> __TDO__CTRL.CTRL.LongitudinalControl/9  "BrakeSwitch[1;3]"
  TDBusSelector/42 -> __TDD__CTRL.CTRL.LongitudinalControl.ClutchPos[0_1]/1  "<ClutchPos[0_1]>"
  __TDD__CTRL.CTRL.LongitudinalControl.ClutchPos[0_1]/1 -> __TDO__CTRL.CTRL.LongitudinalControl/10  "ClutchPos[0_1]"
  TDBusSelector/43 -> __TDD__CTRL.CTRL.LongitudinalControl.DayRunningLight[0;1]/1  "<DayRunningLight[0;1]>"
  __TDD__CTRL.CTRL.LongitudinalControl.DayRunningLight[0;1]/1 -> __TDO__CTRL.CTRL.LongitudinalControl/11  "DayRunningLight[0;1]"
  TDBusSelector/44 -> __TDD__CTRL.CTRL.LongitudinalControl.DriverInfo.ConventionalVehicleSwitch[0;1]/1  "<ConventionalVehicleSwitch[0;1]>"
  __TDD__CTRL.CTRL.LongitudinalControl.DriverInfo.ConventionalVehicleSwitch[0;1]/1 -> __TDO__CTRL.CTRL.LongitudinalControl.DriverInfo/1  "ConventionalVehicleSwitch[0;1]"
  __TDO__CTRL.CTRL.LongitudinalControl.DriverInfo/1 -> __TDO__CTRL.CTRL.LongitudinalControl/12  "DriverInfo"
  TDBusSelector/45 -> __TDD__CTRL.CTRL.LongitudinalControl.DriverInfo.MeanEngDragTrq[Nm]/1  "<MeanEngDragTrq[Nm]>"
  __TDD__CTRL.CTRL.LongitudinalControl.DriverInfo.MeanEngDragTrq[Nm]/1 -> __TDO__CTRL.CTRL.LongitudinalControl.DriverInfo/2  "MeanEngDragTrq[Nm]"
  TDBusSelector/46 -> __TDD__CTRL.CTRL.LongitudinalControl.DriverInfo.MeanEngMaxTrq[Nm]/1  "<MeanEngMaxTrq[Nm]>"
  __TDD__CTRL.CTRL.LongitudinalControl.DriverInfo.MeanEngMaxTrq[Nm]/1 -> __TDO__CTRL.CTRL.LongitudinalControl.DriverInfo/3  "MeanEngMaxTrq[Nm]"
  TDBusSelector/47 -> __TDD__CTRL.CTRL.LongitudinalControl.DriverInfo.ThirtyPercentAccPedalEngTrq[Nm]/1  "<ThirtyPercentAccPedalEngTrq[Nm]>"
  __TDD__CTRL.CTRL.LongitudinalControl.DriverInfo.ThirtyPercentAccPedalEngTrq[Nm]/1 -> __TDO__CTRL.CTRL.LongitudinalControl.DriverInfo/4  "ThirtyPercentAccPedalEngTrq[Nm]"
  __SRC__CTRL.CTRL.LongitudinalControl.DriverInfo.VCUFullAccPedalTrq[Nm]/1 -> __TDO__CTRL.CTRL.LongitudinalControl.DriverInfo/5  "VCUFullAccPedalTrq[Nm]"
  __SRC__CTRL.CTRL.LongitudinalControl.DriverInfo.VCUTorqueRatio[-]/1 -> __TDO__CTRL.CTRL.LongitudinalControl.DriverInfo/6  "VCUTorqueRatio[-]"
  __SRC__CTRL.CTRL.LongitudinalControl.DriverInfo.VCUZeroAccPedalTrq[Nm]/1 -> __TDO__CTRL.CTRL.LongitudinalControl.DriverInfo/7  "VCUZeroAccPedalTrq[Nm]"
  TDBusSelector/48 -> __TDD__CTRL.CTRL.LongitudinalControl.ESCSwitch[0;1]/1  "<ESCSwitch[0;1]>"
  __TDD__CTRL.CTRL.LongitudinalControl.ESCSwitch[0;1]/1 -> __TDO__CTRL.CTRL.LongitudinalControl/13  "ESCSwitch[0;1]"
  TDBusSelector/49 -> __TDD__CTRL.CTRL.LongitudinalControl.EngRunPermission[0;1]/1  "<EngRunPermission[0;1]>"
  __TDD__CTRL.CTRL.LongitudinalControl.EngRunPermission[0;1]/1 -> __TDO__CTRL.CTRL.LongitudinalControl/14  "EngRunPermission[0;1]"
  TDBusSelector/50 -> __TDD__CTRL.CTRL.LongitudinalControl.FogLampFront[0;1]/1  "<FogLampFront[0;1]>"
  __TDD__CTRL.CTRL.LongitudinalControl.FogLampFront[0;1]/1 -> __TDO__CTRL.CTRL.LongitudinalControl/15  "FogLampFront[0;1]"
  TDBusSelector/51 -> __TDD__CTRL.CTRL.LongitudinalControl.FogLampRear[0;1]/1  "<FogLampRear[0;1]>"
  __TDD__CTRL.CTRL.LongitudinalControl.FogLampRear[0;1]/1 -> __TDO__CTRL.CTRL.LongitudinalControl/16  "FogLampRear[0;1]"
  TDBusSelector/52 -> __TDD__CTRL.CTRL.LongitudinalControl.FrontDifferentialLock[0;1]/1  "<FrontDifferentialLock[0;1]>"
  __TDD__CTRL.CTRL.LongitudinalControl.FrontDifferentialLock[0;1]/1 -> __TDO__CTRL.CTRL.LongitudinalControl/17  "FrontDifferentialLock[0;1]"
  TDBusSelector/53 -> __TDD__CTRL.CTRL.LongitudinalControl.FrontLeftWheelBrakePress[Pa]/1  "<FrontLeftWheelBrakePress[Pa]>"
  __TDD__CTRL.CTRL.LongitudinalControl.FrontLeftWheelBrakePress[Pa]/1 -> __TDO__CTRL.CTRL.LongitudinalControl/18  "FrontLeftWheelBrakePress[Pa]"
  TDBusSelector/54 -> __TDD__CTRL.CTRL.LongitudinalControl.FrontRightWheelBrakePress[Pa]/1  "<FrontRightWheelBrakePress[Pa]>"
  __TDD__CTRL.CTRL.LongitudinalControl.FrontRightWheelBrakePress[Pa]/1 -> __TDO__CTRL.CTRL.LongitudinalControl/19  "FrontRightWheelBrakePress[Pa]"
  TDBusSelector/55 -> __TDD__CTRL.CTRL.LongitudinalControl.Handbrake[0_1]/1  "<Handbrake[0_1]>"
  __TDD__CTRL.CTRL.LongitudinalControl.Handbrake[0_1]/1 -> __TDO__CTRL.CTRL.LongitudinalControl/20  "Handbrake[0_1]"
  TDBusSelector/56 -> __TDD__CTRL.CTRL.LongitudinalControl.HighBeamLight[0;1]/1  "<HighBeamLight[0;1]>"
  __TDD__CTRL.CTRL.LongitudinalControl.HighBeamLight[0;1]/1 -> __TDO__CTRL.CTRL.LongitudinalControl/21  "HighBeamLight[0;1]"
  TDBusSelector/57 -> __TDD__CTRL.CTRL.LongitudinalControl.IgnitionSwitch[0;3]/1  "<IgnitionSwitch[0;3]>"
  __TDD__CTRL.CTRL.LongitudinalControl.IgnitionSwitch[0;3]/1 -> __TDO__CTRL.CTRL.LongitudinalControl/22  "IgnitionSwitch[0;3]"
  TDBusSelector/58 -> __TDD__CTRL.CTRL.LongitudinalControl.InitialEngineSpeed[rad/s]/1  "<InitialEngineSpeed[rad/s]>"
  __TDD__CTRL.CTRL.LongitudinalControl.InitialEngineSpeed[rad/s]/1 -> __TDO__CTRL.CTRL.LongitudinalControl/23  "InitialEngineSpeed[rad/s]"
  TDBusSelector/59 -> __TDD__CTRL.CTRL.LongitudinalControl.InitialGear[-4;20]/1  "<InitialGear[-4;20]>"
  __TDD__CTRL.CTRL.LongitudinalControl.InitialGear[-4;20]/1 -> __TDO__CTRL.CTRL.LongitudinalControl/24  "InitialGear[-4;20]"
  TDBusSelector/60 -> __TDD__CTRL.CTRL.LongitudinalControl.InitialSpeed[m/s]/1  "<InitialSpeed[m/s]>"
  __TDD__CTRL.CTRL.LongitudinalControl.InitialSpeed[m/s]/1 -> __TDO__CTRL.CTRL.LongitudinalControl/25  "InitialSpeed[m/s]"
  TDBusSelector/61 -> __TDD__CTRL.CTRL.LongitudinalControl.IntendedEngTrqActive[0;1]/1  "<IntendedEngTrqActive[0;1]>"
  __TDD__CTRL.CTRL.LongitudinalControl.IntendedEngTrqActive[0;1]/1 -> __TDO__CTRL.CTRL.LongitudinalControl/26  "IntendedEngTrqActive[0;1]"
  TDBusSelector/62 -> __TDD__CTRL.CTRL.LongitudinalControl.IntendedEngTrq[Nm]/1  "<IntendedEngTrq[Nm]>"
  __TDD__CTRL.CTRL.LongitudinalControl.IntendedEngTrq[Nm]/1 -> __TDO__CTRL.CTRL.LongitudinalControl/27  "IntendedEngTrq[Nm]"
  TDBusSelector/63 -> __TDD__CTRL.CTRL.LongitudinalControl.KickdownSwitch[0;1]/1  "<KickdownSwitch[0;1]>"
  __TDD__CTRL.CTRL.LongitudinalControl.KickdownSwitch[0;1]/1 -> __TDO__CTRL.CTRL.LongitudinalControl/28  "KickdownSwitch[0;1]"
  TDBusSelector/64 -> __TDD__CTRL.CTRL.LongitudinalControl.LongitudinalPhase[-]/1  "<LongitudinalPhase[-]>"
  __TDD__CTRL.CTRL.LongitudinalControl.LongitudinalPhase[-]/1 -> __TDO__CTRL.CTRL.LongitudinalControl/29  "LongitudinalPhase[-]"
  TDBusSelector/65 -> __TDD__CTRL.CTRL.LongitudinalControl.LowBeamLight[0;1]/1  "<LowBeamLight[0;1]>"
  __TDD__CTRL.CTRL.LongitudinalControl.LowBeamLight[0;1]/1 -> __TDO__CTRL.CTRL.LongitudinalControl/30  "LowBeamLight[0;1]"
  TDBusSelector/66 -> __TDD__CTRL.CTRL.LongitudinalControl.MSRRequestSwitch[0;2]/1  "<MSRRequestSwitch[0;2]>"
  __TDD__CTRL.CTRL.LongitudinalControl.MSRRequestSwitch[0;2]/1 -> __TDO__CTRL.CTRL.LongitudinalControl/31  "MSRRequestSwitch[0;2]"
  TDBusSelector/67 -> __TDD__CTRL.CTRL.LongitudinalControl.MSRTrq[Nm]/1  "<MSRTrq[Nm]>"
  __TDD__CTRL.CTRL.LongitudinalControl.MSRTrq[Nm]/1 -> __TDO__CTRL.CTRL.LongitudinalControl/32  "MSRTrq[Nm]"
  TDBusSelector/68 -> __TDD__CTRL.CTRL.LongitudinalControl.MainBrakePress[Pa]/1  "<MainBrakePress[Pa]>"
  __TDD__CTRL.CTRL.LongitudinalControl.MainBrakePress[Pa]/1 -> __TDO__CTRL.CTRL.LongitudinalControl/33  "MainBrakePress[Pa]"
  TDBusSelector/69 -> __TDD__CTRL.CTRL.LongitudinalControl.ManualGear[-4;20]/1  "<ManualGear[-4;20]>"
  __TDD__CTRL.CTRL.LongitudinalControl.ManualGear[-4;20]/1 -> __TDO__CTRL.CTRL.LongitudinalControl/34  "ManualGear[-4;20]"
  TDBusSelector/70 -> __TDD__CTRL.CTRL.LongitudinalControl.MaxGear[-4;20]/1  "<MaxGear[-4;20]>"
  __TDD__CTRL.CTRL.LongitudinalControl.MaxGear[-4;20]/1 -> __TDO__CTRL.CTRL.LongitudinalControl/35  "MaxGear[-4;20]"
  TDBusSelector/71 -> __TDD__CTRL.CTRL.LongitudinalControl.MinGear[-4;20]/1  "<MinGear[-4;20]>"
  __TDD__CTRL.CTRL.LongitudinalControl.MinGear[-4;20]/1 -> __TDO__CTRL.CTRL.LongitudinalControl/36  "MinGear[-4;20]"
  TDBusSelector/72 -> __TDD__CTRL.CTRL.LongitudinalControl.ParkingLock[0;1]/1  "<ParkingLock[0;1]>"
  __TDD__CTRL.CTRL.LongitudinalControl.ParkingLock[0;1]/1 -> __TDO__CTRL.CTRL.LongitudinalControl/37  "ParkingLock[0;1]"
  TDBusSelector/73 -> __TDD__CTRL.CTRL.LongitudinalControl.Rear2DifferentialLock[0;1]/1  "<Rear2DifferentialLock[0;1]>"
  __TDD__CTRL.CTRL.LongitudinalControl.Rear2DifferentialLock[0;1]/1 -> __TDO__CTRL.CTRL.LongitudinalControl/38  "Rear2DifferentialLock[0;1]"
  TDBusSelector/74 -> __TDD__CTRL.CTRL.LongitudinalControl.Rear2LeftWheelBrakePress[Pa]/1  "<Rear2LeftWheelBrakePress[Pa]>"
  __TDD__CTRL.CTRL.LongitudinalControl.Rear2LeftWheelBrakePress[Pa]/1 -> __TDO__CTRL.CTRL.LongitudinalControl/39  "Rear2LeftWheelBrakePress[Pa]"
  TDBusSelector/75 -> __TDD__CTRL.CTRL.LongitudinalControl.Rear2RightWheelBrakePress[Pa]/1  "<Rear2RightWheelBrakePress[Pa]>"
  __TDD__CTRL.CTRL.LongitudinalControl.Rear2RightWheelBrakePress[Pa]/1 -> __TDO__CTRL.CTRL.LongitudinalControl/40  "Rear2RightWheelBrakePress[Pa]"
  TDBusSelector/76 -> __TDD__CTRL.CTRL.LongitudinalControl.Rear3DifferentialLock[0;1]/1  "<Rear3DifferentialLock[0;1]>"
  __TDD__CTRL.CTRL.LongitudinalControl.Rear3DifferentialLock[0;1]/1 -> __TDO__CTRL.CTRL.LongitudinalControl/41  "Rear3DifferentialLock[0;1]"
  TDBusSelector/77 -> __TDD__CTRL.CTRL.LongitudinalControl.Rear3LeftWheelBrakePress[Pa]/1  "<Rear3LeftWheelBrakePress[Pa]>"
  __TDD__CTRL.CTRL.LongitudinalControl.Rear3LeftWheelBrakePress[Pa]/1 -> __TDO__CTRL.CTRL.LongitudinalControl/42  "Rear3LeftWheelBrakePress[Pa]"
  TDBusSelector/78 -> __TDD__CTRL.CTRL.LongitudinalControl.Rear3RightWheelBrakePress[Pa]/1  "<Rear3RightWheelBrakePress[Pa]>"
  __TDD__CTRL.CTRL.LongitudinalControl.Rear3RightWheelBrakePress[Pa]/1 -> __TDO__CTRL.CTRL.LongitudinalControl/43  "Rear3RightWheelBrakePress[Pa]"
  TDBusSelector/79 -> __TDD__CTRL.CTRL.LongitudinalControl.RearDifferentialLock[0;1]/1  "<RearDifferentialLock[0;1]>"
  __TDD__CTRL.CTRL.LongitudinalControl.RearDifferentialLock[0;1]/1 -> __TDO__CTRL.CTRL.LongitudinalControl/44  "RearDifferentialLock[0;1]"
  TDBusSelector/80 -> __TDD__CTRL.CTRL.LongitudinalControl.RearLeftWheelBrakePress[Pa]/1  "<RearLeftWheelBrakePress[Pa]>"
  __TDD__CTRL.CTRL.LongitudinalControl.RearLeftWheelBrakePress[Pa]/1 -> __TDO__CTRL.CTRL.LongitudinalControl/45  "RearLeftWheelBrakePress[Pa]"
  TDBusSelector/81 -> __TDD__CTRL.CTRL.LongitudinalControl.RearRightWheelBrakePress[Pa]/1  "<RearRightWheelBrakePress[Pa]>"
  __TDD__CTRL.CTRL.LongitudinalControl.RearRightWheelBrakePress[Pa]/1 -> __TDO__CTRL.CTRL.LongitudinalControl/46  "RearRightWheelBrakePress[Pa]"
  __SRC__CTRL.CTRL.LongitudinalControl.RefAccEnforced/1 -> __TDO__CTRL.CTRL.LongitudinalControl/47  "RefAccEnforced"
  __SRC__CTRL.CTRL.LongitudinalControl.RefAcc[m/s**2]/1 -> __TDO__CTRL.CTRL.LongitudinalControl/48  "RefAcc[m/s**2]"
  __SRC__CTRL.CTRL.LongitudinalControl.RefSpdEnforced/1 -> __TDO__CTRL.CTRL.LongitudinalControl/49  "RefSpdEnforced"
  __SRC__CTRL.CTRL.LongitudinalControl.RefSpd[m/s]/1 -> __TDO__CTRL.CTRL.LongitudinalControl/50  "RefSpd[m/s]"
  TDBusSelector/82 -> __TDD__CTRL.CTRL.LongitudinalControl.ShiftingProgramSelection[-]/1  "<ShiftingProgramSelection[-]>"
  __TDD__CTRL.CTRL.LongitudinalControl.ShiftingProgramSelection[-]/1 -> __TDO__CTRL.CTRL.LongitudinalControl/51  "ShiftingProgramSelection[-]"
  TDBusSelector/83 -> __TDD__CTRL.CTRL.LongitudinalControl.StarterSwitch[0;1]/1  "<StarterSwitch[0;1]>"
  __TDD__CTRL.CTRL.LongitudinalControl.StarterSwitch[0;1]/1 -> __TDO__CTRL.CTRL.LongitudinalControl/52  "StarterSwitch[0;1]"
  TDBusSelector/84 -> __TDD__CTRL.CTRL.LongitudinalControl.TrailerFrontLeftWheelBrakePress[Pa]/1  "<TrailerFrontLeftWheelBrakePress[Pa]>"
  __TDD__CTRL.CTRL.LongitudinalControl.TrailerFrontLeftWheelBrakePress[Pa]/1 -> __TDO__CTRL.CTRL.LongitudinalControl/53  "TrailerFrontLeftWheelBrakePress[Pa]"
  TDBusSelector/85 -> __TDD__CTRL.CTRL.LongitudinalControl.TrailerFrontRightWheelBrakePress[Pa]/1  "<TrailerFrontRightWheelBrakePress[Pa]>"
  __TDD__CTRL.CTRL.LongitudinalControl.TrailerFrontRightWheelBrakePress[Pa]/1 -> __TDO__CTRL.CTRL.LongitudinalControl/54  "TrailerFrontRightWheelBrakePress[Pa]"
  TDBusSelector/86 -> __TDD__CTRL.CTRL.LongitudinalControl.TrailerRear2LeftWheelBrakePress[Pa]/1  "<TrailerRear2LeftWheelBrakePress[Pa]>"
  __TDD__CTRL.CTRL.LongitudinalControl.TrailerRear2LeftWheelBrakePress[Pa]/1 -> __TDO__CTRL.CTRL.LongitudinalControl/55  "TrailerRear2LeftWheelBrakePress[Pa]"
  TDBusSelector/87 -> __TDD__CTRL.CTRL.LongitudinalControl.TrailerRear2RightWheelBrakePress[Pa]/1  "<TrailerRear2RightWheelBrakePress[Pa]>"
  __TDD__CTRL.CTRL.LongitudinalControl.TrailerRear2RightWheelBrakePress[Pa]/1 -> __TDO__CTRL.CTRL.LongitudinalControl/56  "TrailerRear2RightWheelBrakePress[Pa]"
  TDBusSelector/88 -> __TDD__CTRL.CTRL.LongitudinalControl.TrailerRear3LeftWheelBrakePress[Pa]/1  "<TrailerRear3LeftWheelBrakePress[Pa]>"
  __TDD__CTRL.CTRL.LongitudinalControl.TrailerRear3LeftWheelBrakePress[Pa]/1 -> __TDO__CTRL.CTRL.LongitudinalControl/57  "TrailerRear3LeftWheelBrakePress[Pa]"
  TDBusSelector/89 -> __TDD__CTRL.CTRL.LongitudinalControl.TrailerRear3RightWheelBrakePress[Pa]/1  "<TrailerRear3RightWheelBrakePress[Pa]>"
  __TDD__CTRL.CTRL.LongitudinalControl.TrailerRear3RightWheelBrakePress[Pa]/1 -> __TDO__CTRL.CTRL.LongitudinalControl/58  "TrailerRear3RightWheelBrakePress[Pa]"
  TDBusSelector/90 -> __TDD__CTRL.CTRL.LongitudinalControl.TrailerRearLeftWheelBrakePress[Pa]/1  "<TrailerRearLeftWheelBrakePress[Pa]>"
  __TDD__CTRL.CTRL.LongitudinalControl.TrailerRearLeftWheelBrakePress[Pa]/1 -> __TDO__CTRL.CTRL.LongitudinalControl/59  "TrailerRearLeftWheelBrakePress[Pa]"
  TDBusSelector/91 -> __TDD__CTRL.CTRL.LongitudinalControl.TrailerRearRightWheelBrakePress[Pa]/1  "<TrailerRearRightWheelBrakePress[Pa]>"
  __TDD__CTRL.CTRL.LongitudinalControl.TrailerRearRightWheelBrakePress[Pa]/1 -> __TDO__CTRL.CTRL.LongitudinalControl/60  "TrailerRearRightWheelBrakePress[Pa]"
  TDBusSelector/92 -> __TDD__CTRL.CTRL.LongitudinalControl.TransferCaseLock[0;1]/1  "<TransferCaseLock[0;1]>"
  __TDD__CTRL.CTRL.LongitudinalControl.TransferCaseLock[0;1]/1 -> __TDO__CTRL.CTRL.LongitudinalControl/61  "TransferCaseLock[0;1]"
  TDBusSelector/93 -> __TDD__CTRL.CTRL.LongitudinalControl.TransmissionLoad[0_1]/1  "<TransmissionLoad[0_1]>"
  __TDD__CTRL.CTRL.LongitudinalControl.TransmissionLoad[0_1]/1 -> __TDO__CTRL.CTRL.LongitudinalControl/62  "TransmissionLoad[0_1]"
  __SRC__CTRL.CTRL.LongitudinalControl.UserDefinedRefValueEnforced/1 -> __TDO__CTRL.CTRL.LongitudinalControl/63  "UserDefinedRefValueEnforced"
  __SRC__CTRL.CTRL.LongitudinalControl.UserDefinedRefValue[-]/1 -> __TDO__CTRL.CTRL.LongitudinalControl/64  "UserDefinedRefValue[-]"
  TDBusSelector/94 -> __TDD__CTRL.CTRL.LongitudinalControl.VCUIntendedMainBrakePressActive[0;1]/1  "<IntendedMainBrakePressActive[0;1]>"
  __TDD__CTRL.CTRL.LongitudinalControl.VCUIntendedMainBrakePressActive[0;1]/1 -> __TDO__CTRL.CTRL.LongitudinalControl/65  "VCUIntendedMainBrakePressActive[0;1]"
  TDBusSelector/95 -> __TDD__CTRL.CTRL.LongitudinalControl.VCUIntendedMainBrakePress[Pa]/1  "<IntendedMainBrakePress[Pa]>"
  __TDD__CTRL.CTRL.LongitudinalControl.VCUIntendedMainBrakePress[Pa]/1 -> __TDO__CTRL.CTRL.LongitudinalControl/66  "VCUIntendedMainBrakePress[Pa]"
  __SRC__CTRL.CTRL.TireCondition.FrontLeftRelInflPress[Pa]/1 -> __TDO__CTRL.CTRL.TireCondition/1  "FrontLeftRelInflPress[Pa]"
  __TDO__CTRL.CTRL.TireCondition/1 -> __TDO__CTRL.CTRL/6  "TireCondition"
  __SRC__CTRL.CTRL.TireCondition.FrontRightRelInflPress[Pa]/1 -> __TDO__CTRL.CTRL.TireCondition/2  "FrontRightRelInflPress[Pa]"
  __SRC__CTRL.CTRL.TireCondition.RearLeftRelInflPress[Pa]/1 -> __TDO__CTRL.CTRL.TireCondition/3  "RearLeftRelInflPress[Pa]"
  __SRC__CTRL.CTRL.TireCondition.RearRightRelInflPress[Pa]/1 -> __TDO__CTRL.CTRL.TireCondition/4  "RearRightRelInflPress[Pa]"
  __SRC__CTRL.CTRL.UserDefinedPhaseTermination.UserDefinedPhaseTermination10[-]/1 -> __TDO__CTRL.CTRL.UserDefinedPhaseTermination/1  "UserDefinedPhaseTermination10[-]"
  __TDO__CTRL.CTRL.UserDefinedPhaseTermination/1 -> __TDO__CTRL.CTRL/7  "UserDefinedPhaseTermination"
  __SRC__CTRL.CTRL.UserDefinedPhaseTermination.UserDefinedPhaseTermination1[-]/1 -> __TDO__CTRL.CTRL.UserDefinedPhaseTermination/2  "UserDefinedPhaseTermination1[-]"
  __SRC__CTRL.CTRL.UserDefinedPhaseTermination.UserDefinedPhaseTermination2[-]/1 -> __TDO__CTRL.CTRL.UserDefinedPhaseTermination/3  "UserDefinedPhaseTermination2[-]"
  __SRC__CTRL.CTRL.UserDefinedPhaseTermination.UserDefinedPhaseTermination3[-]/1 -> __TDO__CTRL.CTRL.UserDefinedPhaseTermination/4  "UserDefinedPhaseTermination3[-]"
  __SRC__CTRL.CTRL.UserDefinedPhaseTermination.UserDefinedPhaseTermination4[-]/1 -> __TDO__CTRL.CTRL.UserDefinedPhaseTermination/5  "UserDefinedPhaseTermination4[-]"
  __SRC__CTRL.CTRL.UserDefinedPhaseTermination.UserDefinedPhaseTermination5[-]/1 -> __TDO__CTRL.CTRL.UserDefinedPhaseTermination/6  "UserDefinedPhaseTermination5[-]"
  __SRC__CTRL.CTRL.UserDefinedPhaseTermination.UserDefinedPhaseTermination6[-]/1 -> __TDO__CTRL.CTRL.UserDefinedPhaseTermination/7  "UserDefinedPhaseTermination6[-]"
  __SRC__CTRL.CTRL.UserDefinedPhaseTermination.UserDefinedPhaseTermination7[-]/1 -> __TDO__CTRL.CTRL.UserDefinedPhaseTermination/8  "UserDefinedPhaseTermination7[-]"
  __SRC__CTRL.CTRL.UserDefinedPhaseTermination.UserDefinedPhaseTermination8[-]/1 -> __TDO__CTRL.CTRL.UserDefinedPhaseTermination/9  "UserDefinedPhaseTermination8[-]"
  __SRC__CTRL.CTRL.UserDefinedPhaseTermination.UserDefinedPhaseTermination9[-]/1 -> __TDO__CTRL.CTRL.UserDefinedPhaseTermination/10  "UserDefinedPhaseTermination9[-]"
  TDBusSelector/96 -> __TDD__CTRL.CTRL.VehicleLights.BrakeLightState[0;1]/1  "<BrakeLightState[0;1]>"
  __TDD__CTRL.CTRL.VehicleLights.BrakeLightState[0;1]/1 -> __TDO__CTRL.CTRL.VehicleLights/1  "BrakeLightState[0;1]"
  __TDO__CTRL.CTRL.VehicleLights/1 -> __TDO__CTRL.CTRL/8  "VehicleLights"
  TDBusSelector/97 -> __TDD__CTRL.CTRL.VehicleLights.DayRunningLightState[0;1]/1  "<DayRunningLightState[0;1]>"
  __TDD__CTRL.CTRL.VehicleLights.DayRunningLightState[0;1]/1 -> __TDO__CTRL.CTRL.VehicleLights/2  "DayRunningLightState[0;1]"
  TDBusSelector/98 -> __TDD__CTRL.CTRL.VehicleLights.FogLampFrontState[0;1]/1  "<FogLampFrontState[0;1]>"
  __TDD__CTRL.CTRL.VehicleLights.FogLampFrontState[0;1]/1 -> __TDO__CTRL.CTRL.VehicleLights/3  "FogLampFrontState[0;1]"
  TDBusSelector/99 -> __TDD__CTRL.CTRL.VehicleLights.FogLampRearState[0;1]/1  "<FogLampRearState[0;1]>"
  __TDD__CTRL.CTRL.VehicleLights.FogLampRearState[0;1]/1 -> __TDO__CTRL.CTRL.VehicleLights/4  "FogLampRearState[0;1]"
  TDBusSelector/100 -> __TDD__CTRL.CTRL.VehicleLights.HighBeamLightState[0;1]/1  "<HighBeamLightState[0;1]>"
  __TDD__CTRL.CTRL.VehicleLights.HighBeamLightState[0;1]/1 -> __TDO__CTRL.CTRL.VehicleLights/5  "HighBeamLightState[0;1]"
  TDBusSelector/101 -> __TDD__CTRL.CTRL.VehicleLights.LeftIndicatorState[0;1]/1  "<LeftIndicatorState[0;1]>"
  __TDD__CTRL.CTRL.VehicleLights.LeftIndicatorState[0;1]/1 -> __TDO__CTRL.CTRL.VehicleLights/6  "LeftIndicatorState[0;1]"
  TDBusSelector/102 -> __TDD__CTRL.CTRL.VehicleLights.LowBeamLightState[0;1]/1  "<LowBeamLightState[0;1]>"
  __TDD__CTRL.CTRL.VehicleLights.LowBeamLightState[0;1]/1 -> __TDO__CTRL.CTRL.VehicleLights/7  "LowBeamLightState[0;1]"
  TDBusSelector/103 -> __TDD__CTRL.CTRL.VehicleLights.ReversingLampState[0;1]/1  "<ReversingLampState[0;1]>"
  __TDD__CTRL.CTRL.VehicleLights.ReversingLampState[0;1]/1 -> __TDO__CTRL.CTRL.VehicleLights/8  "ReversingLampState[0;1]"
  TDBusSelector/104 -> __TDD__CTRL.CTRL.VehicleLights.RightIndicatorState[0;1]/1  "<RightIndicatorState[0;1]>"
  __TDD__CTRL.CTRL.VehicleLights.RightIndicatorState[0;1]/1 -> __TDO__CTRL.CTRL.VehicleLights/9  "RightIndicatorState[0;1]"
  __TDO__CTRL/1 -> CTRL___UNIQUE_1/1  "CTRL"
